simulink model "VCU_SW"  (R2020b)
settings: Solver=FixedStepDiscrete  StartTime=0.0  StopTime=inf  FixedStep=1e-2  RelTol=1e-3
PreLoadFcn:
  | RTWConfigurationCB('preloadfcn', bdroot);
InitFcn:
  | loadvar_ttc500
undefined symbols (not defined in the file): BrkPedalTypes, CabMovModeTypes, cFuseTempSensAcc_X, cFuseTempSensAcc_Y, cFuseTempSensVal_X, cFuseTempSensVal_Y, cTMSTempSensVal_X, cTMSTempSensVal_Y, cTransferCaseSpeedRatio, diag_state, DoorsPositionTypes, dP_filter_Y, DriverOccClassSystemTypes, ErrorValueTypes, fatal_error_callback, IO_ADC_NO_RANGE, LadderStatusTypes, pAnalogCabRotSensAcc, pAnalogCabRotSensMaxVolt, pAnalogCabRotSensMinVolt, pAnalogCabRotSensRange, pAnalogCabRotSensZeroVolt, pBrkActivePress, pCabTiltSensAcc, pCabTiltSensMaxCur, pCabTiltSensMinCur, pDistanceCorrection, pECANManual_BPNEnable, pECANManual_BPNEnabler_Flag, pFilterSensAccRes, pHDirMaxDiffFrq, pHDirSensHighLvl, pHDirSensLowLvl, pMainGearRatio, pMaxFilterSensRes, pMaxFirstPedalSensValue, pMaxFuseTempSensRes, pMaxPressLoss, pMaxPressSensCurrent, pMaxPressValue, pMaxPressValueHydMotAndPump, pMaxPressValueParkDrain, pMaxSecondPedalSensValue, pMaxTempSensVoltage, pMaxTempValue, pMaxTMSTempSensRes, pMinFilterSensRes, pMinFirstPedalSensValue, pMinFuseTempSensRes, pMinPressLoss, pMinPressSensCurrent, pMinPressValue, pMinSecondPedalSensValue, pMinTempSensVoltage, pMinTempValue, pMinTMSTempSensRes, pMotorRingTeethNum, pPedalSensAccuracyPct, pPedalSensAccuracyVolt, pPressLossTreshhold ... (+20)
libraries: TTlibrary x270, canmsglib x127, simulink x88
(part 1 of 17)
settings Model: Creator=Muravev  LastModifiedBy=pirozhkov
settings DataIOCC: ReturnWorkspaceOutputs=off
settings OptimizationCC: DefaultParameterBehavior=Inlined  DefaultUnderspecifiedDataType=single  EnhancedBackFolding=on  PassReuseOutputArgsAs=Individual arguments  OptimizeBlockOrder=speed  DifferentSizesBufferReuse=on  OptimizationCustomize=off  EfficientTunableParamExpr=on
settings DebuggingCC: ParameterTunabilityLossMsg=error  UnitsInconsistencyMsg=none
settings HardwareCC: ProdBitPerPointer=32  ProdBitPerSizeT=32  ProdBitPerPtrDiffT=32  ProdLargestAtomicInteger=Long  ProdLargestAtomicFloat=Double  ProdEndianess=BigEndian  ProdWordSize=32  ProdHWDeviceType=Texas Instruments->TMS570 Cortex-R4
settings ModelReferenceCC: PropagateSignalLabelsOutOfModel=off
settings SFSimCC: SimCustomHeaderCode="#include \"swcAppEnumTypes.h\""  SimUserIncludeDirs="\"C:\\Users\\muravev\\Desktop\\DumperSoftware\\classes\""  MATLABDynamicMemAlloc=off
settings RTWCC: Description=TTcontrol  SystemTargetFile=ttc_500_series.tlc  GenCodeOnly=on  GenerateMakefile=off  TemplateMakefile=ttc_500_series_tmf  GenerateReport=on  LaunchReport=on
settings RTWCC: CustomHeaderCode=|
  | #include "swcAppEnumTypes.h"
  | #include "IO_CAN.h"
settings CodeAppCC: ForceParamTrailComments=on  IgnoreCustomStorageClasses=off  OperatorAnnotations=on  SimulinkDataObjDesc=on  SFDataObjDesc=on  InsertBlockDesc=on
settings STFCustomTargetCC: TargetLangStandard=C99 (ISO)  MultiwordLength=256  ConcurrentExecutionCompliant=off  CombineOutputUpdateFcns=on  ERTCustomFileBanners=on  SupportContinuousTime=off  SupportNonInlinedSFcns=off  RemoveResetFunc=on  MATLABClassNameForMDSCustomization=Simulink.SoftwareTarget.ERTCustomization  CPPClassGenCompliant=off  GRTInterface=off  SystemTargetFile=ttc_500_series.tlc
settings ERTTargetCC: TargetLangStandard=C99 (ISO)  ParMdlRefBuildCompliant=off  CompOptLevelCompliant=off  ConcurrentExecutionCompliant=off  ModelStepFunctionPrototypeControlCompliant=off  CPPClassGenCompliant=off  UseToolchainInfoCompliant=off  InlinedParameterPlacement=NonHierarchical  ERTCustomFileTemplate=ttc_500_series_main.tlc  EnableUserReplacementTypes=on  MaxIdUint32=UBYTE4_MAX_VALUE  MinIdInt16=UBYTE2_MAX_VALUE  MaxIdUint8=UBYTE1_MAX_VALUE  BooleanTrueId=TT_TRUE  BooleanFalseId=TT_FALSE  TypeLimitIdReplacementHeaderFile=ptypes_tms570

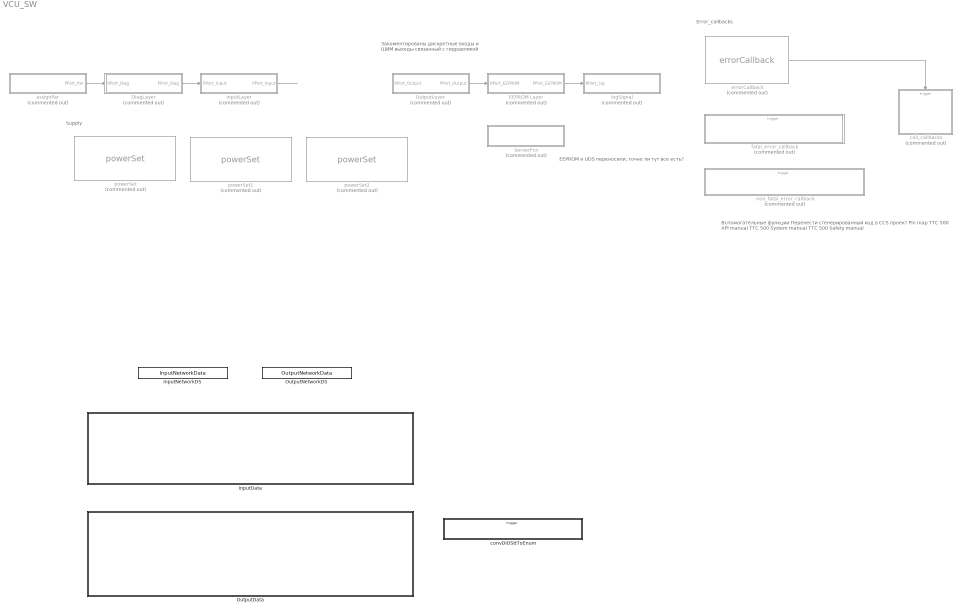
== system VCU_SW ==
  note: EEPROM и UDS переносили, точно ли тут все есть?
  note: Закоментированы дискретные входы
      | и ШИМ выходы связанный с гидравликой
  note: Supply
  note: Error_callbacks
  note: Вспомогательные функции
      |
      | Перенести сгенерированный код в CCS проект
      |
      | Pin map
      |
      | TTC 500 API manual
      |
      | TTC 500 System manual
      |
      | TTC 500 Safety manual
  DiagLayer : Subsystem  Tag=diagnostic layer  Priority=2  Commented=on  TreatAsAtomicUnit=on
      settings: RTWSystemCode=Nonreusable function
  EEPROM Layer : Subsystem  Tag=application layer  Priority=4  Commented=on  TreatAsAtomicUnit=on
      settings: RTWSystemCode=Nonreusable function
  InputData : Subsystem
  InputLayer : Subsystem  Tag=input interface layer  Priority=3  Commented=on  TreatAsAtomicUnit=on
      settings: RTWSystemCode=Nonreusable function
  InputNetworkDS : DataStoreMemory  DataStoreName=InputNetworkData  ReadBeforeWriteMsg=warning  WriteAfterWriteMsg=warning  WriteAfterReadMsg=warning  ShowAdditionalParam=off  OutDataTypeStr=Bus: CANInputStruct
  OutputData : Subsystem
  OutputLayer : Subsystem  Tag=output interface layer  Priority=5  Commented=on  TreatAsAtomicUnit=on
      settings: RTWSystemCode=Nonreusable function
  OutputNetworkDS : DataStoreMemory  DataStoreName=OutputNetworkData  ReadBeforeWriteMsg=warning  WriteAfterWriteMsg=warning  WriteAfterReadMsg=warning  ShowAdditionalParam=off  OutDataTypeStr=Bus: CANOutputStruct
  ServerFcn : Subsystem  Commented=on
  assignPar : Subsystem  Priority=1  Commented=on  TreatAsAtomicUnit=on
      settings: RTWSystemCode=Nonreusable function
  call_callbacks : Subsystem  Commented=on  TreatAsAtomicUnit=on
  convDIOSttToEnum : Subsystem  TreatAsAtomicUnit=on
  errorCallback : TTlibrary/DIAG/errorCallback  Commented=on  SFunctionModules=''
      settings: SourceProductName=TT control 500 series
  fatal_error_callback : Subsystem  Commented=on  TreatAsAtomicUnit=on
  logSignal : Subsystem  Priority=6  Commented=on  TreatAsAtomicUnit=on
      settings: RTWSystemCode=Nonreusable function
  non_fatal_error_callback : Subsystem  Commented=on  TreatAsAtomicUnit=on
  powerSet : TTlibrary/POWER/powerSet  Commented=on  pin=IO_SENSOR_SUPPLY_0  mode=IO_POWER_ON  sample_time=-1
      settings: SourceProductName=TT control 500 series
  powerSet1 : TTlibrary/POWER/powerSet  Commented=on  pin=IO_SENSOR_SUPPLY_1  mode=IO_POWER_ON  sample_time=-1
      settings: SourceProductName=TT control 500 series
  powerSet2 : TTlibrary/POWER/powerSet  Commented=on  pin=IO_SENSOR_SUPPLY_2  mode=IO_POWER_ON_5V  sample_time=-1
      settings: SourceProductName=TT control 500 series
  wires:
  DiagLayer/1(PPort_Diag) -> InputLayer/1(RPort_Input)
  ? -> OutputLayer/1(RPort_Output)
  errorCallback/1 -> call_callbacks/Trigger
  assignPar/1(PPort_Par) -> DiagLayer/1(RPort_Diag)
  InputLayer/1(PPort_Input) -> ?
  OutputLayer/1(PPort_Output) -> EEPROM Layer/1(RPort_EEPROM)
  EEPROM Layer/1(PPort_EEPROM) -> logSignal/1(RPort_Sig)

== system VCU_SW/DiagLayer ==
  note: DM1 - 0x13 - Steering
  note: DM1 - 0x00 - Engine
  note: DEM - Diagnostic Event Manager
      | FIM - Function Inhibition Manager
  note: DM1 - 0x5A - Emotor
  note: DM1 - 0x1A - Generator
  RPort_Diag : Inport
  Ground : Ground
  Terminator1 : Terminator
  PPort_Diag : Outport
  wires:
  RPort_Diag/1 -> Terminator1/1
  Ground/1 -> PPort_Diag/1

== system VCU_SW/EEPROM Layer ==
  RPort_EEPROM : Inport
  Data Store Read1 : DataStoreRead  Commented=on  DataStoreName=InputInterfaceData  DataStoreElements=InputInterfaceData.DI.selector_signal_1
  Data Store Read2 : DataStoreRead  Commented=on  DataStoreName=InputInterfaceData  DataStoreElements=InputInterfaceData.DI.selector_signal_2
  Data Store Read3 : DataStoreRead  DataStoreName=InputInterfaceData  DataStoreElements=InputInterfaceData.DI.T15Common
  Data Store Read8 : DataStoreRead  Commented=on  DataStoreName=InputInterfaceData  DataStoreElements=InputInterfaceData.DI.T15Common
  Data Store Write : DataStoreWrite  Commented=on  DataStoreName=InputInterfaceData  DataStoreElements=InputInterfaceData.DI.transCaseHighGearIsActiveSens
  Data Store Write1 : DataStoreWrite  Commented=on  DataStoreName=InputInterfaceData  DataStoreElements=InputInterfaceData.DI.transCaseLowGearIsActiveSens
  Data Store Write2 : DataStoreWrite  DataStoreName=UDSStruct  DataStoreElements=UDSStruct.sucReadFlag
  Data Store Write3 : DataStoreWrite  DataStoreName=UDSStruct  DataStoreElements=UDSStruct.sucWriteFlag
  EEPROM Client : MATLAB Function  TreatAsAtomicUnit=on
  EEPROM Client2 : MATLAB Function  Commented=on  TreatAsAtomicUnit=on
  Function Caller : FunctionCaller  Commented=on  FunctionPrototype=enumValue = convDIOSttToEnum(rawValue,errorSts)  InputArgumentSpecifications=<Enter example>  OutputArgumentSpecifications=<Enter example>
  Function Caller1 : FunctionCaller  Commented=on  FunctionPrototype=enumValue = convDIOSttToEnum(rawValue,errorSts)  InputArgumentSpecifications=<Enter example>  OutputArgumentSpecifications=<Enter example>
  Ground : Ground  Commented=on
  Ground2 : Ground  Commented=on
  Ground3 : Ground  Commented=on
  Simulink Function : Subsystem  Commented=on  TreatAsAtomicUnit=on
  Simulink Function1 : Subsystem  Commented=on  TreatAsAtomicUnit=on
  Simulink Function2 : Subsystem  Commented=on  TreatAsAtomicUnit=on
  Simulink Function3 : Subsystem  Commented=on  TreatAsAtomicUnit=on
  Terminator1 : Terminator  Commented=on
  calculate trip distance : Subsystem  Commented=on
  readProcessing : Subsystem  TreatAsAtomicUnit=on
  updateUDSStruct : Subsystem  TreatAsAtomicUnit=on
  writeProcessing : Subsystem  TreatAsAtomicUnit=on
  PPort_EEPROM : Outport
  wires:
  RPort_EEPROM/1 -> Terminator1/1
  Ground/1 -> PPort_EEPROM/1
  Data Store Read8/1 -> EEPROM Client2/1(t15common)
  Data Store Read1/1 -> EEPROM Client2/2(sig1)
  Data Store Read2/1 -> EEPROM Client2/3(sig2)
  EEPROM Client2/2(write_flag) -> Function Caller/1
  EEPROM Client2/1(read_flag) -> Function Caller1/1
  Function Caller/1 -> Data Store Write1/1
  Function Caller1/1 -> Data Store Write/1
  Ground2/1 -> Function Caller/2
  Ground3/1 -> Function Caller1/2
  Data Store Read3/1 -> EEPROM Client/1(t15common)
  EEPROM Client/1(sucReadFlag) -> Data Store Write2/1
  EEPROM Client/2(sucWriteFlag) -> Data Store Write3/1

== system VCU_SW/InputData ==
  InputData : Subsystem
  Pin101_Pin104_CMD_fa : Subsystem

== system VCU_SW/InputLayer ==
  note: Helper Fcns
  RPort_Input : Inport
  Ground1 : Ground  Commented=on
  InputInterfaces : Subsystem  Tag=input interface layer  Priority=2  Commented=on  TreatAsAtomicUnit=on
      settings: RTWSystemCode=Nonreusable function
  InputNetwork : Subsystem  Tag=input interface layer  Priority=3  Commented=on  TreatAsAtomicUnit=on
      settings: RTWSystemCode=Nonreusable function
  InputTimers : Subsystem  Commented=on  TreatAsAtomicUnit=on
  Manual : Subsystem  Commented=on  TreatAsAtomicUnit=on
  Simulink Function : Subsystem  Commented=on  TreatAsAtomicUnit=on
  Simulink Function1 : Subsystem  Commented=on  TreatAsAtomicUnit=on
  Simulink Function2 : Subsystem  Commented=on  TreatAsAtomicUnit=on
  Terminator5 : Terminator  Commented=on
  currentDOConv : Subsystem  Commented=on  TreatAsAtomicUnit=on
  voltageDOConv : Subsystem  Commented=on  TreatAsAtomicUnit=on
  PPort_Input : Outport
  wires:
  RPort_Input/1 -> Terminator5/1
  Ground1/1 -> PPort_Input/1

== system VCU_SW/OutputData ==
  CANPack_VLVCMD_HYD1 : canmsglib/CAN Pack  CANdbFile=database\TTCTest.dbc  MsgList=Pin101_Pin104_FB  MsgName=Pin101_Pin104_FB  MsgIDType=Extended (29-bit identifier)  MsgIdentifier=419364903  MsgLength=8  Remote=off  ApplyMinMax=off  BusOutput=on  SignalInfo={ 'Pin101_FB', '0', '16', 'LE', 'unsigned', 'Standard', '0', '1', '0', '0', '65535' }
      settings: SourceProductBaseCode=ME,XP,VN  DataFormat=manually specified signals
  Data Store Read : DataStoreRead  DataStoreName=OutputNetworkData  DataStoreElements=OutputNetworkData.Pin101_Pin104_FB.Pin0_feedback
  Terminator1 : Terminator
  transmit_message_vlvcmd_hyd1 : TTlibrary/CAN/transmit_message_name  channel=IO_CAN_CHANNEL_0  id_format=IO_CAN_EXT_FRAME  retranslation=off  io_error=on  sample_time=-1
      settings: SourceProductName=TT control 500 series
  wires:
  transmit_message_vlvcmd_hyd1/1 -> Terminator1/1  "error_tx_transmit_message_vlvcmd_hyd1"
  Data Store Read/1 -> CANPack_VLVCMD_HYD1/1
  CANPack_VLVCMD_HYD1/1 -> transmit_message_vlvcmd_hyd1/1

== system VCU_SW/OutputLayer ==
  RPort_Output : Inport
  Ground1 : Ground
  OutputInterfaces : Subsystem  Tag=input interface layer  Priority=3  TreatAsAtomicUnit=on
      settings: RTWSystemCode=Nonreusable function
  OutputNetwork : Subsystem  Tag=input interface layer  Priority=3  TreatAsAtomicUnit=on
      settings: RTWSystemCode=Nonreusable function
  Terminator5 : Terminator
  PPort_Output : Outport
  wires:
  RPort_Output/1 -> Terminator5/1
  Ground1/1 -> PPort_Output/1

== system VCU_SW/ServerFcn ==
  note: проверить полином
  note: CAN Communication
  note: Diagnostic
  note: Interface
  note: Конвертация типов данных
  Simulink Function : Subsystem  Commented=on  TreatAsAtomicUnit=on
  Simulink Function1 : Subsystem  Commented=on  TreatAsAtomicUnit=on
  Simulink Function2 : Subsystem  Commented=on  TreatAsAtomicUnit=on
  Simulink Function3 : Subsystem  Commented=on  TreatAsAtomicUnit=on
  Simulink Function4 : Subsystem  Commented=on  TreatAsAtomicUnit=on
  calcAbsVal : Subsystem  Commented=on  TreatAsAtomicUnit=on
  calcCRC16 : Subsystem  TreatAsAtomicUnit=on
  calcMaxVal : Subsystem  Commented=on  TreatAsAtomicUnit=on
  calcMinVal : Subsystem  Commented=on  TreatAsAtomicUnit=on
  convAICurrentData : Subsystem  TreatAsAtomicUnit=on
  convAIDiagDataToEnum : Subsystem  Commented=on  TreatAsAtomicUnit=on
  convAIResistanceData : Subsystem  TreatAsAtomicUnit=on
  convAIVoltageData : Subsystem  TreatAsAtomicUnit=on
  convCANDiagDataToEnum : Subsystem  TreatAsAtomicUnit=on
  convDIDiagDataToEnum : Subsystem  Commented=on  TreatAsAtomicUnit=on
  convDIOStatusTypeToNum : Subsystem  TreatAsAtomicUnit=on
  convDIOStsTypeToNum : Subsystem  TreatAsAtomicUnit=on
  convDIOSttToEnum : Subsystem  TreatAsAtomicUnit=on
  convDIOSttTypeToNum : Subsystem  TreatAsAtomicUnit=on
  convDODiagDataToEnum : Subsystem  Commented=on  TreatAsAtomicUnit=on
  convDataStsToEnum : Subsystem  TreatAsAtomicUnit=on
  convDiagDataForTest : Subsystem  TreatAsAtomicUnit=on
  convINint1 : Subsystem  Commented=on  TreatAsAtomicUnit=on
  convINint16 : Subsystem  TreatAsAtomicUnit=on
  convINuint16 : Subsystem  TreatAsAtomicUnit=on
  convPWDData : Subsystem  TreatAsAtomicUnit=on
  convPWDDiagDataToEnum : Subsystem  Commented=on  TreatAsAtomicUnit=on
  convPWMDiagDataToEnum : Subsystem  Commented=on  TreatAsAtomicUnit=on
  convUintPinToenumStt : Subsystem  TreatAsAtomicUnit=on

== system VCU_SW/assignPar ==
  Ground : Ground  Commented=on
  PPort_Par : Outport
  wires:
  Ground/1 -> PPort_Par/1

== system VCU_SW/call_callbacks ==
  function : TriggerPort  TriggerType=function-call  VariantControl=Variant
  Function Caller : FunctionCaller  FunctionPrototype=fatal_error_callback(diag_state,watchdog_state,error)  InputArgumentSpecifications=<Enter example>  OutputArgumentSpecifications=<Enter example>
  Function Caller1 : FunctionCaller  FunctionPrototype=action = non_fatal_error_callback(diag_state,watchdog_state,error)  InputArgumentSpecifications=<Enter example>  OutputArgumentSpecifications=<Enter example>
  Ground{,1..5} (6 alike) : Ground
  Terminator : Terminator
  wires:
  Function Caller1/1 -> Terminator/1
  Ground/1 -> Function Caller1/1
  Ground1/1 -> Function Caller1/2
  Ground2/1 -> Function Caller1/3
  Ground5/1 -> Function Caller/3
  Ground4/1 -> Function Caller/2
  Ground3/1 -> Function Caller/1

== system VCU_SW/convDIOSttToEnum ==
  convDIOSttToEnum : TriggerPort  TriggerType=function-call  IsSimulinkFunction=on  FunctionName=convDIOSttToEnum  VariantControl=(inherit)
  MATLAB Function : MATLAB Function  TreatAsAtomicUnit=on
  rawValue : ArgIn  DisableCoverage=on  OutDataTypeStr=boolean  ArgumentName=rawValue
  errorSts : ArgIn  DisableCoverage=on  Port=2  OutDataTypeStr=uint16  ArgumentName=errorSts
  enumValue : ArgOut  DisableCoverage=on  OutDataTypeStr=Enum: StateModeTypes  ArgumentName=enumValue
  wires:
  MATLAB Function/1(enum) -> enumValue/1
  rawValue/1 -> MATLAB Function/1(value)
  errorSts/1 -> MATLAB Function/2(error)

== system VCU_SW/fatal_error_callback ==
  fatal_error_callback : TriggerPort  TriggerType=function-call  IsSimulinkFunction=on  FunctionName=fatal_error_callback  VariantControl=(inherit)
  Bus Selector1 : BusSelector  OutputSignals=error_code,device_num,faulty_value
  Terminator{1..2,4..6} (5 alike) : Terminator
  diag_state : ArgIn  DisableCoverage=on  OutDataTypeStr=uint8  ArgumentName=diag_state
  watchdog_state : ArgIn  DisableCoverage=on  Port=2  OutDataTypeStr=uint8  ArgumentName=watchdog_state
  error : ArgIn  DisableCoverage=on  Port=3  OutDataTypeStr=Bus: DIAG_ERRORCODE  ArgumentName=error
  wires:
  watchdog_state/1 -> Terminator2/1
  Bus Selector1/1 -> Terminator4/1  "<error_code>"
  Bus Selector1/2 -> Terminator5/1  "<device_num>"
  Bus Selector1/3 -> Terminator6/1  "<faulty_value>"
  diag_state/1 -> Terminator1/1
  error/1 -> Bus Selector1/1

== system VCU_SW/logSignal ==
  RPort_Sig : Inport
  10msec : simulink/Ports & Subsystems/Function-Call Generator  sample_time=0.01  numberOfIterations=1  DisallowWideOutput=off
  Constant : Constant  Value=uint8(0)
  Terminator1 : Terminator
  daqFcn_mf : MATLAB Function  TreatAsAtomicUnit=on
  getDAQCmd : Subsystem  TreatAsAtomicUnit=on
  getListData : Subsystem  TreatAsAtomicUnit=on
  getListNum : Subsystem  TreatAsAtomicUnit=on
  transmitDAQMsg : Subsystem  TreatAsAtomicUnit=on
  wires:
  10msec/1 -> daqFcn_mf/Trigger
  RPort_Sig/1 -> Terminator1/1
  Constant/1 -> daqFcn_mf/1(diagTxEna)

== system VCU_SW/non_fatal_error_callback ==
  note: See IO_PIN.h in API manual
  note: watchdog_state values
      | 1. DIAG_WD_STATE_ACTIVE 0x06U - Watchdog CPU is in active state
      | 2. DIAG_WD_STATE_DIAGNOSTIC 0x05U - Watchdog CPU is in diagnostic state
      | 3. DIAG_WD_STATE_RESET 0x03U - Watchdog CPU is in reset state
      | 4. DIAG_WD_STATE_SAFE 0x09U - Watchdog CPU is in safe state
      | 5. DIAG_WD_STATE_STANDBY 0x01U - Watchdog CPU is in standby state
      | 6. DIAG_WD_STATE_UNKNOWN 0xFFU - Watchdog CPU is in an unknown stat e
  note: diag_state values
      | 1. DIAG_STATE_CONFIG 0x05 - Diagnostic state machine is in config state
      | 2. DIAG_STATE_DISABLED 0x00UL - Diagnostic state machine is disabled
      | 3. DIAG_STATE_INIT 0x03UL - Diagnostic state machine is in init state
      | 4. DIAG_STATE_MAIN 0x06UL - Diagnostic state machine is in main state
      | 5. DIAG_STATE_SAFE 0x09UL - Diagnostic state machine is in safe state
  note: Values for action
      | 1. DIAG_ERR_NOACTION take no action (ignore the error)
      | 2. DIAG_ERR_SAFESTATE enter the safe state (switch off all outputs)
      | 3. DIAG_ERR_DISABLE_SSW0 disable the shut-off group 0 (IO_INT_SAFETY_SW_0)
      | 4. DIAG_ERR_DISABLE_SSW1 disable the shut-off group 1 (IO_INT_SAFETY_SW_1)
      | 5. DIAG_ERR_DISABLE_SSW2 disable the shut-off group 2 (IO_INT_SAFETY_SW_2)
      | 6. DIAG_ERR_DISABLE_HS00 disable the high side digital output 0 (IO_DO_00)
      | 7. DIAG_ERR_DISABLE_HS01 disable the high side digital output 1 (IO_DO_01)
      | 8. DIAG_ERR_DISABLE_HS02 disable the high side digital output 2 (IO_DO_02)
      | 9. DIAG_ERR_DISABLE_HS03 disable the high side digital output 3 (IO_DO_03)
      | 10. DIAG_ERR_DISABLE_HS04 disable the high side digital output 4 (IO_DO_04)
      | 11. DIAG_ERR_DISABLE_HS05 disable the high side digital output 5 (IO_DO_05)
      | 12. DIAG_ERR_DISABLE_HS06 disable the high side digital output 6 (IO_DO_06)
      | 13. DIAG_ERR_DISABLE_HS07 disable the high side digital output 7 (IO_DO_07)
  note: See siagnostic state machine error codes in DIAG_Constants.h API manual
  f : TriggerPort  TriggerType=function-call  IsSimulinkFunction=on  FunctionName=non_fatal_error_callback  VariantControl=(inherit)
  Bus Selector : BusSelector  OutputSignals=error_code,device_num,faulty_value
  Ground : Ground
  Terminator{,1..4} (5 alike) : Terminator
  u : ArgIn  DisableCoverage=on  OutDataTypeStr=uint8  ArgumentName=diag_state
  u1 : ArgIn  DisableCoverage=on  Port=2  OutDataTypeStr=uint8  ArgumentName=watchdog_state
  u2 : ArgIn  DisableCoverage=on  Port=3  OutDataTypeStr=Bus: DIAG_ERRORCODE  ArgumentName=error
  y : ArgOut  DisableCoverage=on  OutDataTypeStr=uint8  ArgumentName=action
  wires:
  Ground/1 -> y/1
  u/1 -> Terminator/1
  u1/1 -> Terminator1/1
  u2/1 -> Bus Selector/1
  Bus Selector/1 -> Terminator2/1  "<error_code>"
  Bus Selector/2 -> Terminator3/1  "<device_num>"
  Bus Selector/3 -> Terminator4/1  "<faulty_value>"

== system VCU_SW/EEPROM Layer/Simulink Function ==
  readProcessing : TriggerPort  TriggerType=function-call  IsSimulinkFunction=on  FunctionName=readProcessing  FunctionVisibility=scoped  VariantControl=(inherit)
  Data Store Write1 : DataStoreWrite  DataStoreName=UDSStruct  DataStoreElements=UDSStruct.read_sts
  eeprom_read_processing_kora : MATLAB Function  TreatAsAtomicUnit=on
  flag : ArgOut  DisableCoverage=on  OutDataTypeStr=boolean  ArgumentName=flag
  wires:
  eeprom_read_processing_kora/1(flag) -> flag/1
  eeprom_read_processing_kora/2(read_sts) -> Data Store Write1/1

== system VCU_SW/EEPROM Layer/Simulink Function1 ==
  writeProcessing : TriggerPort  TriggerType=function-call  IsSimulinkFunction=on  FunctionName=writeProcessing  FunctionVisibility=scoped  VariantControl=(inherit)
  Data Store Write1 : DataStoreWrite  DataStoreName=UDSStruct  DataStoreElements=UDSStruct.write_sts
  eeprom_write_processing_kora : MATLAB Function  TreatAsAtomicUnit=on
  flag : ArgOut  DisableCoverage=on  OutDataTypeStr=boolean  ArgumentName=flag
  wires:
  eeprom_write_processing_kora/1(flag) -> flag/1
  eeprom_write_processing_kora/2(write_sts) -> Data Store Write1/1

== system VCU_SW/EEPROM Layer/Simulink Function2 ==
  setDataToWrite : TriggerPort  TriggerType=function-call  IsSimulinkFunction=on  FunctionName=setDataToWrite  FunctionVisibility=scoped  VariantControl=(inherit)
  Constant : Constant  Value=uint16(1)
  Constant1 : Constant  Value=uint16(2)
  Constant2 : Constant  Value=uint16(3)
  Constant3 : Constant  Value=uint32(4)
  Constant4 : Constant  Value=uint8(5)
  Constant5 : Constant  Value=uint8(6)
  Constant6 : Constant  Value=uint8(7)
  Constant7 : Constant  Value=uint8(8)
  Constant8 : Constant  Value=uint16(9)
  Constant9 : Constant  Value=uint16(10)
  Data Store Write1 : DataStoreWrite  DataStoreName=UDSStruct  DataStoreElements=UDSStruct.DistanceM#UDSStruct.DistanceKM#UDSStruct.DistanceKKM#UDSStruct.EngineHours#UDSStruct.TransPumpVolumeMax#UDSStruct.TransMotorVolumeMin#UDSStruct.AccelerationPedalMaxEngSpd#UDSStruct.AccelerationPedalMinEngSpd#UDSStruct.EngineSpeedMax#UDSStruct.EngineSpeedMin
  wires:
  Constant/1 -> Data Store Write1/1
  Constant1/1 -> Data Store Write1/2
  Constant2/1 -> Data Store Write1/3
  Constant3/1 -> Data Store Write1/4
  Constant4/1 -> Data Store Write1/5
  Constant5/1 -> Data Store Write1/6
  Constant6/1 -> Data Store Write1/7
  Constant7/1 -> Data Store Write1/8
  Constant8/1 -> Data Store Write1/9
  Constant9/1 -> Data Store Write1/10

== system VCU_SW/EEPROM Layer/Simulink Function3 ==
  get_eeprom_status : TriggerPort  TriggerType=function-call  IsSimulinkFunction=on  FunctionName=get_eeprom_status  FunctionVisibility=scoped  VariantControl=(inherit)
  Data Store Write2 : DataStoreWrite  DataStoreName=UDSStruct  DataStoreElements=UDSStruct.eeprom_sts
  eeprom_write_processing_kora : MATLAB Function  TreatAsAtomicUnit=on
  wires:
  eeprom_write_processing_kora/1(eeprom_sts) -> Data Store Write2/1

== system VCU_SW/EEPROM Layer/calculate trip distance ==
  Constant : Constant  Value=pDistanceCorrection
  Constant1 : Constant  Value=uint32(0)
  Data Store Read : DataStoreRead  DataStoreName=EEPROMData  DataStoreElements=EEPROMData.tripDistM
  Data Store Read1 : DataStoreRead  DataStoreName=EEPROMData  DataStoreElements=EEPROMData.tripDistM_Trip
  Data Store Read2 : DataStoreRead  DataStoreName=EEPROMData  DataStoreElements=EEPROMData.Trip_Reset
  Data Store Read8 : DataStoreRead  DataStoreName=InputFunctionsData  DataStoreElements=InputFunctionsData.vehicleSpeed
  Data Store Write : DataStoreWrite  DataStoreName=EEPROMData  DataStoreElements=EEPROMData.tripDistM
  Data Store Write1 : DataStoreWrite  DataStoreName=EEPROMData  DataStoreElements=EEPROMData.tripDistM_Trip
  Display1 : Display
  Display2 : Display
  EEPROM read : Subsystem  TreatAsAtomicUnit=on
      settings: RTWSystemCode=Nonreusable function
  EEPROM read1 : Subsystem  TreatAsAtomicUnit=on
      settings: RTWSystemCode=Nonreusable function
  Enumerated Constant : simulink/Sources/Enumerated Constant  OutDataTypeStr=Enum: StateModeTypes  Value=StateModeTypes.STT_ENABLE  SampleTime=inf
  Equal : RelationalOperator  Operator===  OutDataTypeStr=boolean  RndMeth=Simplest
  Function-Call Split13 : FunctionCallSplit  NumOutputPorts=2
  Multiport Switch : MultiPortSwitch  DataPortOrder=Zero-based contiguous  Inputs=2  zeroidx=on
  Scope : Scope
  Scope1 : Scope  NumInputPorts=2
  Sum : Sum  Inputs=++|
  Sum1 : Sum  Inputs=++|
  calcTotalDistCtrl : MATLAB Function  TreatAsAtomicUnit=on
  calcTripDist : MATLAB Function  TreatAsAtomicUnit=on
  wires:
  Data Store Read8/1 -> calcTripDist/1(vehSpd)  "vehspd"
  Constant/1 -> calcTripDist/2(correction)
  Sum/1 -> EEPROM read/1(In1), Data Store Write/1
  Data Store Read/1 -> Display2/1, Sum/2
  calcTripDist/1(distance) -> Sum1/1, Display1/1, Sum/1, Scope/1
  calcTripDist/2(a) -> Scope1/1  "algo"
  calcTotalDistCtrl/1(calcTotalDist()) -> Function-Call Split13/1
  Data Store Read1/1 -> Sum1/2
  Sum1/1 -> Multiport Switch/2
  Multiport Switch/1 -> EEPROM read1/1(In1), Data Store Write1/1
  Data Store Read2/1 -> Equal/1
  Enumerated Constant/1 -> Equal/2
  Equal/1 -> Multiport Switch/1
  Constant1/1 -> Multiport Switch/3
  Function-Call Split13/1 -> EEPROM read/Trigger
  Function-Call Split13/2 -> EEPROM read1/Trigger

== system VCU_SW/EEPROM Layer/readProcessing ==
  readProcessing : TriggerPort  TriggerType=function-call  IsSimulinkFunction=on  FunctionName=readProcessing  FunctionVisibility=scoped  VariantControl=(inherit)
  eeprom_read_processing_kora : MATLAB Function  TreatAsAtomicUnit=on
  flag : ArgOut  DisableCoverage=on  OutDataTypeStr=boolean  ArgumentName=flag
  wires:
  eeprom_read_processing_kora/1(flag) -> flag/1

== system VCU_SW/EEPROM Layer/updateUDSStruct ==
  updateUDSStruct : TriggerPort  TriggerType=function-call  IsSimulinkFunction=on  FunctionName=updateUDSStruct  FunctionVisibility=scoped  VariantControl=(inherit)
  Data Store Read1 : DataStoreRead  DataStoreName=EngineControllerData  DataStoreElements=EngineControllerData.EngineHours
  Data Store Read5 : DataStoreRead  DataStoreName=InputFunctionsData  DataStoreElements=InputFunctionsData.Distance
  MATLAB Function : MATLAB Function  TreatAsAtomicUnit=on
  MATLAB Function1 : MATLAB Function  TreatAsAtomicUnit=on
  wires:
  Data Store Read5/1 -> MATLAB Function1/1(Distance)
  Data Store Read1/1 -> MATLAB Function/1(EngineHours)

== system VCU_SW/EEPROM Layer/writeProcessing ==
  writeProcessing : TriggerPort  TriggerType=function-call  IsSimulinkFunction=on  FunctionName=writeProcessing  FunctionVisibility=scoped  VariantControl=(inherit)
  eeprom_write_processing_kora : MATLAB Function  TreatAsAtomicUnit=on
  flag : ArgOut  DisableCoverage=on  OutDataTypeStr=boolean  ArgumentName=flag
  wires:
  eeprom_write_processing_kora/1(flag) -> flag/1

== system VCU_SW/InputData/InputData ==
  AnalogInputs : Subsystem
  DigitalInputs : Subsystem

== system VCU_SW/InputData/Pin101_Pin104_CMD_fa ==
  CANUnpack_Pin101_Pin104_CMD : canmsglib/CAN Unpack  CANdbFile=database\TTCTest.dbc  MsgList=Pin101_Pin104_CMD  MsgName=Pin101_Pin104_CMD  MsgIDType=Extended (29-bit identifier)  MsgIdentifier=419365114  MsgLength=8  SignalInfo={ 'Pin101_config', '0', '3', 'LE', 'unsigned', 'Standard', '0', '1', '0', '0', '7'; 'Pin101_value', '8', '8', 'LE', 'unsigned', 'Standard', '0', '1', '0', '0', '100' }  IDPort=off  TimestampPort=off  ErrorPort=off  RemotePort=off  LengthPort=off  StatusPort=off  ApplyMinMax=off
      settings: SourceProductBaseCode=ME,XP,VN
  DataStoreWrite_Str_BJM2 : DataStoreWrite  DataStoreName=InputNetworkData  DataStoreElements=InputNetworkData.Pin101_Pin104_CMD.PinCFG.Pin0_config#InputNetworkData.Pin101_Pin104_CMD.PinCMD.Pin0_value
  Terminator4 : Terminator
  read_message_Pin101_Pin104_CMD : TTlibrary/CAN/read_message_name  channel=IO_CAN_CHANNEL_0  id_format=IO_CAN_EXT_FRAME  get_msg_info=off  message_names=there is no CAN Unpack blocks  message_info=|  id=419365114  ac_mask=536870911  retranslation=off  io_error=on  sample_time=-1
      | Message Name: BJM1
      |  Message ID Type: Extended (29-bit identifier)
      |  Message ID: 419288581
      settings: SourceProductName=TT control 500 series
  wires:
  read_message_Pin101_Pin104_CMD/1 -> CANUnpack_Pin101_Pin104_CMD/1  "msg_419365114"
  read_message_Pin101_Pin104_CMD/2 -> Terminator4/1  "handler_err_419365114"
  CANUnpack_Pin101_Pin104_CMD/1 -> DataStoreWrite_Str_BJM2/1
  CANUnpack_Pin101_Pin104_CMD/2 -> DataStoreWrite_Str_BJM2/2

== system VCU_SW/InputLayer/InputInterfaces ==
  AnalogInput : Subsystem  Tag=input interface layer  Priority=3  TreatAsAtomicUnit=on
      settings: RTWSystemCode=Nonreusable function
  DigitalInput : Subsystem  Tag=input interface layer  Priority=3  TreatAsAtomicUnit=on
      settings: RTWSystemCode=Nonreusable function
  PWDInput : Subsystem  Tag=input interface layer  Priority=3  TreatAsAtomicUnit=on
      settings: RTWSystemCode=Nonreusable function
  PWMCurrentInput : Subsystem  Tag=input interface layer  Priority=3  TreatAsAtomicUnit=on
      settings: RTWSystemCode=Nonreusable function

== system VCU_SW/InputLayer/InputNetwork ==
  note: Здесь
  note: Каналы CAN:
      | - Hyd-CAN 0
      | - C-CAN 1
      | - Engine-CAN 2
      | - Str-CAN 3
      | - ----- 4
      | - xCrane-CAN 5
      | - Diag-CAN 6
  InputCCAN : Subsystem  Tag=input interface layer  Priority=3  TreatAsAtomicUnit=on
      settings: RTWSystemCode=Nonreusable function
  InputDiagCAN : Subsystem  Tag=input interface layer  Priority=3  TreatAsAtomicUnit=on
      settings: RTWSystemCode=Nonreusable function
  InputEngCAN : Subsystem  Tag=input interface layer  Priority=3  TreatAsAtomicUnit=on
      settings: RTWSystemCode=Nonreusable function
  InputHydCAN : Subsystem  Tag=input interface layer  Priority=3  TreatAsAtomicUnit=on
      settings: RTWSystemCode=Nonreusable function
  InputStrCAN : Subsystem  Tag=input interface layer  Priority=3  TreatAsAtomicUnit=on
      settings: RTWSystemCode=Nonreusable function
  InputxCraneCAN : Subsystem  Tag=input interface layer  Priority=3  TreatAsAtomicUnit=on
      settings: RTWSystemCode=Nonreusable function

== system VCU_SW/InputLayer/InputTimers ==
  1000msec : simulink/Ports & Subsystems/Function-Call Generator  Commented=on  sample_time=1  numberOfIterations=1  DisallowWideOutput=off
  100msec : simulink/Ports & Subsystems/Function-Call Generator  Commented=on  sample_time=0.1  numberOfIterations=1  DisallowWideOutput=off
  10msec : simulink/Ports & Subsystems/Function-Call Generator  Commented=on  sample_time=0.01  numberOfIterations=1  DisallowWideOutput=off
  MATLAB Function : MATLAB Function  Commented=on  TreatAsAtomicUnit=on
  MATLAB Function1 : MATLAB Function  Commented=on  TreatAsAtomicUnit=on
  MATLAB Function2 : MATLAB Function  Commented=on  TreatAsAtomicUnit=on
  wires:
  1000msec/1 -> MATLAB Function2/Trigger
  100msec/1 -> MATLAB Function1/Trigger
  10msec/1 -> MATLAB Function/Trigger

== system VCU_SW/InputLayer/Manual ==
  100msec : simulink/Ports & Subsystems/Function-Call Generator  sample_time=0.1  numberOfIterations=1  DisallowWideOutput=off
  GetManual : Subsystem  TreatAsAtomicUnit=on
      settings: RTWSystemCode=Nonreusable function
  wires:
  100msec/1 -> GetManual/Trigger

== system VCU_SW/InputLayer/Simulink Function ==
  currentPWMConv : TriggerPort  TriggerType=function-call  IsSimulinkFunction=on  FunctionName=currentPWMConv  FunctionVisibility=scoped  VariantControl=(inherit)
  Constant : Constant  Value=single(1000)
  Data Type Conversion : DataTypeConversion  OutDataTypeStr=single
  Divide : Product  Inputs=*/
  rawCur : ArgIn  DisableCoverage=on  OutDataTypeStr=uint16  ArgumentName=rawCur
  finalCur : ArgOut  DisableCoverage=on  OutDataTypeStr=single  ArgumentName=finalCur
  wires:
  Divide/1 -> finalCur/1
  Constant/1 -> Divide/2
  Data Type Conversion/1 -> Divide/1
  rawCur/1 -> Data Type Conversion/1

== system VCU_SW/InputLayer/Simulink Function1 ==
  convPWMCurrData : TriggerPort  TriggerType=function-call  IsSimulinkFunction=on  FunctionName=convPWMCurrData  FunctionVisibility=scoped  VariantControl=(inherit)
  MATLAB Function : MATLAB Function  TreatAsAtomicUnit=on
  rawValue : ArgIn  OutDataTypeStr=uint16  ArgumentName=rawValue
  errorSts : ArgIn  Port=2  OutDataTypeStr=uint16  ArgumentName=errorSts
  finalValue : ArgOut  DisableCoverage=on  OutDataTypeStr=uint16  ArgumentName=finalValue
  wires:
  MATLAB Function/1(outValue) -> finalValue/1
  rawValue/1 -> MATLAB Function/1(inpValue)
  errorSts/1 -> MATLAB Function/2(errorSts)

== system VCU_SW/InputLayer/Simulink Function2 ==
  voltageAIConv : TriggerPort  TriggerType=function-call  IsSimulinkFunction=on  FunctionName=voltageAIConv  FunctionVisibility=scoped  VariantControl=(inherit)
  Constant : Constant  Value=pVoltageTreshold
  MATLAB Function : MATLAB Function  TreatAsAtomicUnit=on
  Volt : ArgIn  DisableCoverage=on  OutDataTypeStr=uint16  ArgumentName=Volt
  finalState : ArgOut  DisableCoverage=on  OutDataTypeStr=Enum: StateModeTypes  ArgumentName=finalState
  wires:
  Volt/1 -> MATLAB Function/1(volt)
  MATLAB Function/1(state) -> finalState/1
  Constant/1 -> MATLAB Function/2(treshold)

== system VCU_SW/InputLayer/currentDOConv ==
  currentDOConv : TriggerPort  TriggerType=function-call  IsSimulinkFunction=on  FunctionName=currentDOConv  FunctionVisibility=scoped  VariantControl=(inherit)
  Constant : Constant  Value=single(1000)
  Data Type Conversion : DataTypeConversion  OutDataTypeStr=single
  Divide : Product  Inputs=*/
  rawCur : ArgIn  DisableCoverage=on  OutDataTypeStr=uint16  ArgumentName=rawCur
  finalCur : ArgOut  DisableCoverage=on  OutDataTypeStr=single  ArgumentName=finalCur
  wires:
  Divide/1 -> finalCur/1
  Constant/1 -> Divide/2
  Data Type Conversion/1 -> Divide/1
  rawCur/1 -> Data Type Conversion/1

== system VCU_SW/InputLayer/voltageDOConv ==
  voltageDOConv : TriggerPort  TriggerType=function-call  IsSimulinkFunction=on  FunctionName=voltageDOConv  FunctionVisibility=scoped  VariantControl=(inherit)
  Constant : Constant  Value=single(1000)
  Data Type Conversion : DataTypeConversion  OutDataTypeStr=single
  Divide : Product  Inputs=*/
  rawVolt : ArgIn  DisableCoverage=on  OutDataTypeStr=uint16  ArgumentName=rawVolt
  finalVolt : ArgOut  DisableCoverage=on  OutDataTypeStr=single  ArgumentName=finalVolt
  wires:
  rawVolt/1 -> Data Type Conversion/1
  Data Type Conversion/1 -> Divide/1
  Constant/1 -> Divide/2
  Divide/1 -> finalVolt/1

== system VCU_SW/OutputLayer/OutputInterfaces ==
  note: Запасная закомментирована
  note: Закомментирована гидравлика:
      | - тормоза
      | - раздатка
      | - блокировки дифференциалов
      | - тормоз кабины
  DigitalOutput1 : Subsystem  Tag=input interface layer  Priority=3  TreatAsAtomicUnit=on
      settings: RTWSystemCode=Nonreusable function
  PWMOutput : Subsystem  Tag=input interface layer  Priority=3  TreatAsAtomicUnit=on
      settings: RTWSystemCode=Nonreusable function
  exDigitalOutput : Subsystem  Tag=input interface layer  Priority=3  Commented=on  TreatAsAtomicUnit=on
      settings: RTWSystemCode=Nonreusable function

== system VCU_SW/OutputLayer/OutputNetwork ==
  note: Каналы CAN:
      | - Hyd-CAN 0
      | - C-CAN 1
      | - Engine-CAN 2
      | - Str-CAN 3
      | - ----- 4
      | - xCrane-CAN 5
      | - Diag-CAN 6
  OutputCCAN : Subsystem  Tag=input interface layer  Priority=3  TreatAsAtomicUnit=on
      settings: RTWSystemCode=Nonreusable function
  OutputDiagCAN + Logger : Subsystem  Tag=input interface layer  Priority=3  TreatAsAtomicUnit=on
      settings: RTWSystemCode=Nonreusable function
  OutputEngCAN : Subsystem  Tag=input interface layer  Priority=3  TreatAsAtomicUnit=on
      settings: RTWSystemCode=Nonreusable function
  OutputHydCAN : Subsystem  Tag=input interface layer  Priority=3  TreatAsAtomicUnit=on
      settings: RTWSystemCode=Nonreusable function
  OutputStrCAN : Subsystem  Tag=input interface layer  Priority=3  TreatAsAtomicUnit=on
      settings: RTWSystemCode=Nonreusable function
  OutputxCraneCAN : Subsystem  Tag=input interface layer  Priority=3  Commented=on  TreatAsAtomicUnit=on
      settings: RTWSystemCode=Nonreusable function

== system VCU_SW/ServerFcn/Simulink Function ==
  txRequestMsg : TriggerPort  TriggerType=function-call  IsSimulinkFunction=on  FunctionName=txRequestMsg  FunctionVisibility=scoped  VariantControl=(inherit)
  PGN : ArgIn  DisableCoverage=on  ArgumentName=PGN
  DA : ArgIn  Port=2  ArgumentName=DA
  wires:
  PGN/1 -> ?

== system VCU_SW/ServerFcn/Simulink Function1 ==
  rxRequestMsg : TriggerPort  TriggerType=function-call  IsSimulinkFunction=on  FunctionName=rxRequestMsg  FunctionVisibility=scoped  VariantControl=(inherit)
  MsgData : ArgIn  DisableCoverage=on  ArgumentName=MsgData
  ID : ArgIn  Port=2  ArgumentName=ID
  wires:
  MsgData/1 -> ?

== system VCU_SW/ServerFcn/Simulink Function2 ==
  rxAckMsg : TriggerPort  TriggerType=function-call  IsSimulinkFunction=on  FunctionName=rxAckMsg  FunctionVisibility=scoped  VariantControl=(inherit)
  MsgData : ArgIn  DisableCoverage=on  ArgumentName=MsgData
  ID : ArgIn  Port=2  ArgumentName=ID
  wires:
  MsgData/1 -> ?

== system VCU_SW/ServerFcn/Simulink Function3 ==
  rxAckMsg : TriggerPort  TriggerType=function-call  IsSimulinkFunction=on  FunctionName=rxAckMsg  FunctionVisibility=scoped  VariantControl=(inherit)
  MsgData : ArgIn  DisableCoverage=on  ArgumentName=MsgData
  ID : ArgIn  Port=2  ArgumentName=ID
  wires:
  MsgData/1 -> ?

== system VCU_SW/ServerFcn/Simulink Function4 ==
  rxAckMsg : TriggerPort  TriggerType=function-call  IsSimulinkFunction=on  FunctionName=rxAckMsg  FunctionVisibility=scoped  VariantControl=(inherit)
  MsgData : ArgIn  DisableCoverage=on  ArgumentName=MsgData
  ID : ArgIn  Port=2  ArgumentName=ID
  wires:
  MsgData/1 -> ?

== system VCU_SW/ServerFcn/calcAbsVal ==
  note: because fuck matlab, that's why
  calcAbsVal : TriggerPort  TriggerType=function-call  IsSimulinkFunction=on  FunctionName=calcAbsVal  VariantControl=(inherit)
  Constant : Constant  Value=single(0)
  Constant1 : Constant  Value=single(-1)
  MATLAB Function : MATLAB Function  Commented=on  TreatAsAtomicUnit=on
  Multiport Switch : MultiPortSwitch  DataPortOrder=Zero-based contiguous  Inputs=2  zeroidx=on
  Product : Product
  Relational Operator1 : RelationalOperator  Operator=>  OutDataTypeStr='uint8'  RndMeth=Simplest
  rawVal : ArgIn  DisableCoverage=on  OutDataTypeStr=single  ArgumentName=rawVal
  modVal : ArgOut  DisableCoverage=on  OutDataTypeStr=single  ArgumentName=modVal
  wires:
  Relational Operator1/1 -> Multiport Switch/1
  Multiport Switch/1 -> modVal/1
  rawVal/1 -> Relational Operator1/1, Multiport Switch/3, Product/1
  Constant/1 -> Relational Operator1/2
  Product/1 -> Multiport Switch/2
  Constant1/1 -> Product/2

== system VCU_SW/ServerFcn/calcCRC16 ==
  calcCRC16 : TriggerPort  TriggerType=function-call  IsSimulinkFunction=on  FunctionName=calcCRC16  VariantControl=(inherit)
  Data Type Conversion : DataTypeConversion  OutDataTypeStr=uint16
  MATLAB Function : MATLAB Function  TreatAsAtomicUnit=on
  packet : ArgIn  DisableCoverage=on  OutDataTypeStr=uint8  PortDimensions=[1, 6]  ArgumentName=packet
  CRC16 : ArgOut  DisableCoverage=on  OutDataTypeStr=uint16  ArgumentName=CRC16
  wires:
  MATLAB Function/1(crcfinal) -> CRC16/1
  packet/1 -> Data Type Conversion/1
  Data Type Conversion/1 -> MATLAB Function/1(packet)

== system VCU_SW/ServerFcn/calcMaxVal ==
  note: because fuck matlab, that's why
  calcMaxVal : TriggerPort  TriggerType=function-call  IsSimulinkFunction=on  FunctionName=calcMaxVal  VariantControl=(inherit)
  MATLAB Function : MATLAB Function  Commented=on  TreatAsAtomicUnit=on
  Multiport Switch : MultiPortSwitch  DataPortOrder=Zero-based contiguous  Inputs=2  zeroidx=on
  Relational Operator : RelationalOperator  Operator=>  OutDataTypeStr='uint8'  RndMeth=Simplest
  fstVal : ArgIn  DisableCoverage=on  OutDataTypeStr=single  ArgumentName=fstVal
  secVal : ArgIn  Port=2  OutDataTypeStr=single  ArgumentName=secVal
  maxVal : ArgOut  DisableCoverage=on  OutDataTypeStr=single  ArgumentName=maxVal
  wires:
  Multiport Switch/1 -> maxVal/1
  fstVal/1 -> Multiport Switch/3, Relational Operator/1
  secVal/1 -> Multiport Switch/2, Relational Operator/2
  Relational Operator/1 -> Multiport Switch/1

== system VCU_SW/ServerFcn/calcMinVal ==
  note: because fuck matlab, that's why
  calcMinVal : TriggerPort  TriggerType=function-call  IsSimulinkFunction=on  FunctionName=calcMinVal  VariantControl=(inherit)
  MATLAB Function : MATLAB Function  Commented=on  TreatAsAtomicUnit=on
  Multiport Switch : MultiPortSwitch  DataPortOrder=Zero-based contiguous  Inputs=2  zeroidx=on
  Relational Operator : RelationalOperator  Operator=<  OutDataTypeStr='uint8'  RndMeth=Simplest
  fstVal : ArgIn  DisableCoverage=on  OutDataTypeStr=single  ArgumentName=fstVal
  secVal : ArgIn  Port=2  OutDataTypeStr=single  ArgumentName=secVal
  minVal : ArgOut  DisableCoverage=on  OutDataTypeStr=single  ArgumentName=minVal
  wires:
  fstVal/1 -> Relational Operator/1, Multiport Switch/3
  Multiport Switch/1 -> minVal/1
  Relational Operator/1 -> Multiport Switch/1
  secVal/1 -> Multiport Switch/2, Relational Operator/2

== system VCU_SW/ServerFcn/convAICurrentData ==
  convAICurrentData : TriggerPort  TriggerType=function-call  IsSimulinkFunction=on  FunctionName=convAICurrentData  VariantControl=(inherit)
  MATLAB Function : MATLAB Function  TreatAsAtomicUnit=on
  rawValue : ArgIn  OutDataTypeStr=uint32  ArgumentName=rawValue
  errorSts : ArgIn  Port=2  OutDataTypeStr=uint16  ArgumentName=errorSts
  finalValue : ArgOut  DisableCoverage=on  OutDataTypeStr=uint16  ArgumentName=finalValue
  wires:
  rawValue/1 -> MATLAB Function/1(inpValue)
  errorSts/1 -> MATLAB Function/2(errorSts)
  MATLAB Function/1(outValue) -> finalValue/1

== system VCU_SW/ServerFcn/convAIDiagDataToEnum ==
  convAIDiagDataToEnum : TriggerPort  TriggerType=function-call  IsSimulinkFunction=on  FunctionName=convAIDiagDataToEnum  VariantControl=(inherit)
  Ground : Ground
  Terminator : Terminator
  rawValue : ArgIn  DisableCoverage=on  OutDataTypeStr=uint16  ArgumentName=rawValue
  enumValue : ArgOut  DisableCoverage=on  OutDataTypeStr=Enum: DigitalPinStatusTypes  ArgumentName=enumValue
  wires:
  rawValue/1 -> Terminator/1
  Ground/1 -> enumValue/1

== system VCU_SW/ServerFcn/convAIResistanceData ==
  convAIResistanceData : TriggerPort  TriggerType=function-call  IsSimulinkFunction=on  FunctionName=convAIResistanceData  VariantControl=(inherit)
  MATLAB Function : MATLAB Function  TreatAsAtomicUnit=on
  rawValue~ : ArgIn  DisableCoverage=on  OutDataTypeStr=uint32  ArgumentName=rawValue
  errorSts : ArgIn  Port=2  OutDataTypeStr=uint16  ArgumentName=errorSts
  finalValue : ArgOut  DisableCoverage=on  OutDataTypeStr=uint32  ArgumentName=finalValue
  wires:
  MATLAB Function/1(outValue) -> finalValue/1
  rawValue~/1 -> MATLAB Function/1(inpValue)
  errorSts/1 -> MATLAB Function/2(errorSts)

== system VCU_SW/ServerFcn/convAIVoltageData ==
  convAIVoltageData : TriggerPort  TriggerType=function-call  IsSimulinkFunction=on  FunctionName=convAIVoltageData  VariantControl=(inherit)
  MATLAB Function : MATLAB Function  TreatAsAtomicUnit=on
  rawValue : ArgIn  DisableCoverage=on  OutDataTypeStr=uint32  ArgumentName=rawValue
  errorSts : ArgIn  Port=2  OutDataTypeStr=uint16  ArgumentName=errorSts
  finalValue : ArgOut  DisableCoverage=on  OutDataTypeStr=uint16  ArgumentName=finalValue
  wires:
  rawValue/1 -> MATLAB Function/1(inpValue)
  MATLAB Function/1(outValue) -> finalValue/1
  errorSts/1 -> MATLAB Function/2(errorSts)

== system VCU_SW/ServerFcn/convCANDiagDataToEnum ==
  convCANDiagDataToEnum : TriggerPort  TriggerType=function-call  IsSimulinkFunction=on  FunctionName=convCANDiagDataToEnum  VariantControl=(inherit)
  Ground : Ground
  Terminator : Terminator
  rawValue : ArgIn  DisableCoverage=on  OutDataTypeStr=uint16  ArgumentName=rawValue
  enumValue : ArgOut  DisableCoverage=on  OutDataTypeStr=Enum: DigitalPinStatusTypes  ArgumentName=enumValue
  wires:
  rawValue/1 -> Terminator/1
  Ground/1 -> enumValue/1

== system VCU_SW/ServerFcn/convDIDiagDataToEnum ==
  convDIDiagDataToEnum : TriggerPort  TriggerType=function-call  IsSimulinkFunction=on  FunctionName=convDIDiagDataToEnum  VariantControl=(inherit)
  Ground : Ground
  Terminator : Terminator
  rawValue : ArgIn  DisableCoverage=on  OutDataTypeStr=uint16  ArgumentName=rawValue
  enumValue : ArgOut  DisableCoverage=on  OutDataTypeStr=Enum: DigitalPinStatusTypes  ArgumentName=enumValue
  wires:
  rawValue/1 -> Terminator/1
  Ground/1 -> enumValue/1

== system VCU_SW/ServerFcn/convDIOStatusTypeToNum ==
  convDIOStatusTypeToNum : TriggerPort  TriggerType=function-call  IsSimulinkFunction=on  FunctionName=convDIOStatusTypeToNum  VariantControl=(inherit)
  MATLAB Function : MATLAB Function  TreatAsAtomicUnit=on
  enumValue : ArgIn  DisableCoverage=on  OutDataTypeStr=Enum: StatusModeTypes  ArgumentName=enumValue
  rawValue : ArgOut  DisableCoverage=on  OutDataTypeStr=boolean  ArgumentName=rawValue
  wires:
  enumValue/1 -> MATLAB Function/1(enum)
  MATLAB Function/1(value) -> rawValue/1

== system VCU_SW/ServerFcn/convDIOStsTypeToNum ==
  convDIOStsTypeToNum : TriggerPort  TriggerType=function-call  IsSimulinkFunction=on  FunctionName=convDIOStsTypeToNum  VariantControl=(inherit)
  MATLAB Function : MATLAB Function  TreatAsAtomicUnit=on
  enumValue : ArgIn  DisableCoverage=on  OutDataTypeStr=Enum: StateModeTypes  ArgumentName=enumValue
  rawValue : ArgOut  DisableCoverage=on  OutDataTypeStr=boolean  ArgumentName=rawValue
  wires:
  enumValue/1 -> MATLAB Function/1(enum)
  MATLAB Function/1(value) -> rawValue/1

== system VCU_SW/ServerFcn/convDIOSttToEnum ==
  convDIOSttToEnum : TriggerPort  TriggerType=function-call  IsSimulinkFunction=on  FunctionName=convDIOSttToEnum  VariantControl=(inherit)
  MATLAB Function : MATLAB Function  TreatAsAtomicUnit=on
  rawValue : ArgIn  DisableCoverage=on  OutDataTypeStr=boolean  ArgumentName=rawValue
  errorSts : ArgIn  DisableCoverage=on  Port=2  OutDataTypeStr=uint16  ArgumentName=errorSts
  enumValue : ArgOut  DisableCoverage=on  OutDataTypeStr=Enum: StateModeTypes  ArgumentName=enumValue
  wires:
  MATLAB Function/1(enum) -> enumValue/1
  rawValue/1 -> MATLAB Function/1(value)
  errorSts/1 -> MATLAB Function/2(error)

== system VCU_SW/ServerFcn/convDIOSttTypeToNum ==
  convDIOSttTypeToNum : TriggerPort  TriggerType=function-call  IsSimulinkFunction=on  FunctionName=convDIOSttTypeToNum  VariantControl=(inherit)
  MATLAB Function : MATLAB Function  TreatAsAtomicUnit=on
  enumValue : ArgIn  DisableCoverage=on  OutDataTypeStr=Enum: StateModeTypes  ArgumentName=enumValue
  rawValue : ArgOut  DisableCoverage=on  OutDataTypeStr=uint8  ArgumentName=rawValue
  wires:
  enumValue/1 -> MATLAB Function/1(enum)
  MATLAB Function/1(value) -> rawValue/1

== system VCU_SW/ServerFcn/convDODiagDataToEnum ==
  convDODiagDataToEnum : TriggerPort  TriggerType=function-call  IsSimulinkFunction=on  FunctionName=convDODiagDataToEnum  VariantControl=(inherit)
  Ground : Ground
  Terminator : Terminator
  rawValue : ArgIn  DisableCoverage=on  OutDataTypeStr=uint16  ArgumentName=rawValue
  enumValue : ArgOut  DisableCoverage=on  OutDataTypeStr=Enum: DigitalPinStatusTypes  ArgumentName=enumValue
  wires:
  Ground/1 -> enumValue/1
  rawValue/1 -> Terminator/1

== system VCU_SW/ServerFcn/convDataStsToEnum ==
  convDataStsToEnum : TriggerPort  TriggerType=function-call  IsSimulinkFunction=on  FunctionName=convDataStsToEnum  VariantControl=(inherit)
  MATLAB Function : MATLAB Function  TreatAsAtomicUnit=on
  rawValue : ArgIn  DisableCoverage=on  OutDataTypeStr=uint8  ArgumentName=rawValue
  enumValue : ArgOut  DisableCoverage=on  OutDataTypeStr=Enum: StatusModeTypes  ArgumentName=enumValue
  wires:
  rawValue/1 -> MATLAB Function/1(value)
  MATLAB Function/1(enum) -> enumValue/1

== system VCU_SW/ServerFcn/convDiagDataForTest ==
  convDiagDataForTest : TriggerPort  TriggerType=function-call  IsSimulinkFunction=on  FunctionName=convDiagDataForTest  VariantControl=(inherit)
  MATLAB Function : MATLAB Function  TreatAsAtomicUnit=on
  rawValue : ArgIn  DisableCoverage=on  OutDataTypeStr=uint16  ArgumentName=rawValue
  finalValue : ArgOut  DisableCoverage=on  OutDataTypeStr=uint8  ArgumentName=finalValue
  wires:
  MATLAB Function/1(canDiag) -> finalValue/1
  rawValue/1 -> MATLAB Function/1(hwDiag)

== system VCU_SW/ServerFcn/convINint1 ==
  convINint16fromUint16 : TriggerPort  TriggerType=function-call  IsSimulinkFunction=on  FunctionName=convINint16fromUint16  VariantControl=(inherit)
  MATLAB Function2 : MATLAB Function  TreatAsAtomicUnit=on
  x : ArgIn  DisableCoverage=on  OutDataTypeStr=int16  ArgumentName=x
  y : ArgOut  DisableCoverage=on  OutDataTypeStr=int16  ArgumentName=y
  wires:
  MATLAB Function2/1(y) -> y/1
  x/1 -> MATLAB Function2/1(x)

== system VCU_SW/ServerFcn/convINint16 ==
  convINint16 : TriggerPort  TriggerType=function-call  IsSimulinkFunction=on  FunctionName=convINint16  VariantControl=(inherit)
  MATLAB Function2 : MATLAB Function  TreatAsAtomicUnit=on
  x : ArgIn  DisableCoverage=on  OutDataTypeStr=single  ArgumentName=x
  y : ArgOut  DisableCoverage=on  OutDataTypeStr=int16  ArgumentName=y
  wires:
  MATLAB Function2/1(y) -> y/1
  x/1 -> MATLAB Function2/1(x)
